simulink model "simulinkprueba_processing"  (R2018a)
settings: Solver=VariableStepAuto  StartTime=0.0  StopTime=200  RelTol=1e-3
libraries: simulink x1
settings Model: Creator=quich  LastModifiedBy=quich

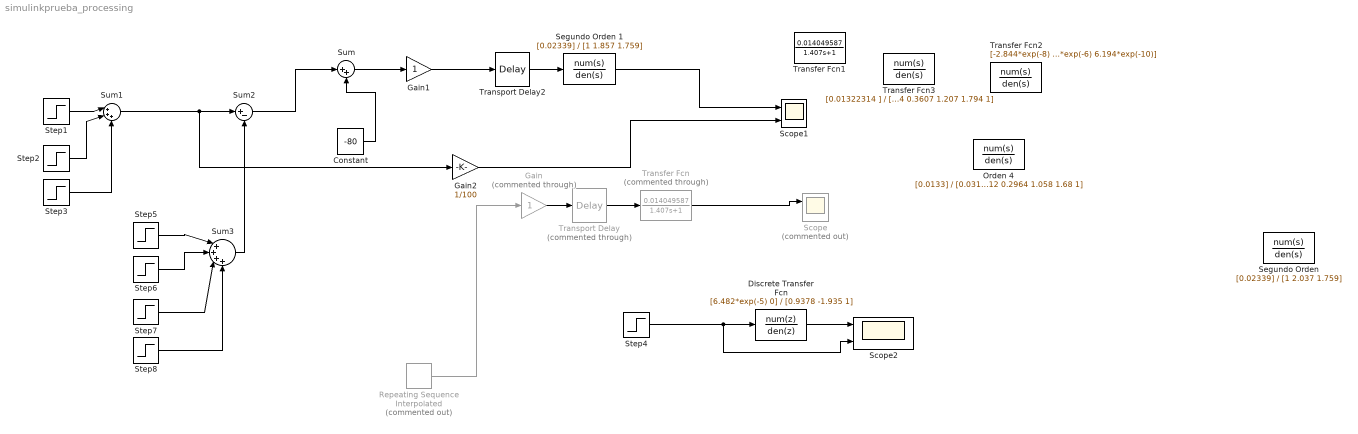
== system simulinkprueba_processing ==
  Constant : Constant  Value=-80  SampleTime=0.055
  Discrete Transfer Fcn : DiscreteTransferFcn  Numerator=[6.482*exp(-5) 0]  Denominator=[0.9378 -1.935 1]  SampleTime=0.055
  Gain : Gain  Commented=through
  Gain1 : Gain
  Gain2 : Gain  Gain=1/100
  "Orden 4 " : TransferFcn  Numerator=[0.0133]  Denominator=[0.03112 0.2964 1.058 1.68 1]
  Repeating Sequence Interpolated : simulink/Sources/Repeating Sequence Interpolated  Commented=on  OutValues=[0 0 100 100 193 193 314 314].'  TimeValues=[0 5 5.01 15 15.01 30 30.01 45].'  LookUpMeth=Interpolation-Use End Values  tsamp=0.01  OutMin=[]  OutMax=[]  OutDataTypeStr=double  OutputDataTypeScalingMode=double  OutDataType=fixdt(0,8)  OutScaling=2^-10
  Scope : Scope  Commented=on  NumInputPorts=2
  Scope1 : Scope  NumInputPorts=2
  Scope2 : Scope  NumInputPorts=2
  "Segundo Orden " : TransferFcn  Numerator=[0.02339]  Denominator=[1 2.037 1.759]
  Segundo Orden 1 : TransferFcn  Numerator=[0.02339]  Denominator=[1 1.857 1.759]
  Step1 : Step  Time=20  Before=100  After=350  SampleTime=0
  Step2 : Step  Time=35  Before=350  After=776  SampleTime=0
  Step3 : Step  Time=70  After=0  SampleTime=0
  Step4 : Step  Time=20  SampleTime=0
  Step5 : Step  Time=55  After=276  SampleTime=0
  Step6 : Step  Time=70  After=500  SampleTime=0
  Step7 : Step  Time=120  After=0  SampleTime=0
  Step8 : Step  Time=140  After=0  SampleTime=0
  Sum : Sum  Inputs=|++
  Sum1 : Sum  Inputs=|+++
  Sum2 : Sum  Inputs=|+-
  Sum3 : Sum  Inputs=|++++
  Transfer Fcn : TransferFcn  Commented=through  Numerator=|  Denominator=|
      Numerator=|
      | [0.014049587
      | ]
      Denominator=|
      | [1.407
      |  1]
  Transfer Fcn1 : TransferFcn  Numerator=|  Denominator=|
      Numerator=|
      | [0.014049587
      | ]
      Denominator=|
      | [1.407
      |  1]
  Transfer Fcn2 : TransferFcn  Numerator=|  Denominator=[1 0.001075 1.316*exp(-6) 6.194*exp(-10)]
      | [-2.844*exp(-8) 1.55*exp(-11)
      | ]
  Transfer Fcn3 : TransferFcn  Numerator=|  Denominator=[0.04044 0.3607 1.207 1.794 1]
      | [0.01322314
      | ]
  Transport Delay : TransportDelay  Commented=through  DelayTime=0.64
  Transport Delay2 : TransportDelay  DelayTime=0.6
  wires:
  Transfer Fcn/1 -> Scope/1
  Transport Delay/1 -> Transfer Fcn/1
  Gain/1 -> Transport Delay/1
  Repeating Sequence Interpolated/1 -> Gain/1
  Gain1/1 -> Transport Delay2/1
  Sum/1 -> Gain1/1
  Step1/1 -> Sum1/1
  Step2/1 -> Sum1/2
  Step3/1 -> Sum1/3
  Sum2/1 -> Sum/1
  Step4/1 -> Scope2/2, Discrete Transfer Fcn/1
  Discrete Transfer Fcn/1 -> Scope2/1
  Sum1/1 -> Gain2/1, Sum2/1
  Gain2/1 -> Scope1/2
  Constant/1 -> Sum/2
  Transport Delay2/1 -> Segundo Orden 1/1
  Segundo Orden 1/1 -> Scope1/1
  Sum3/1 -> Sum2/2
  Step5/1 -> Sum3/1
  Step6/1 -> Sum3/2
  Step7/1 -> Sum3/3
  Step8/1 -> Sum3/4
